simulink model "excercise1_tf2"  (R2023b)
settings: Solver=VariableStepAuto  StartTime=0.0  StopTime=100  RelTol=1e-3
undefined symbols (not defined in the file): d, m
settings Model: Creator=elliot  LastModifiedBy=elliot

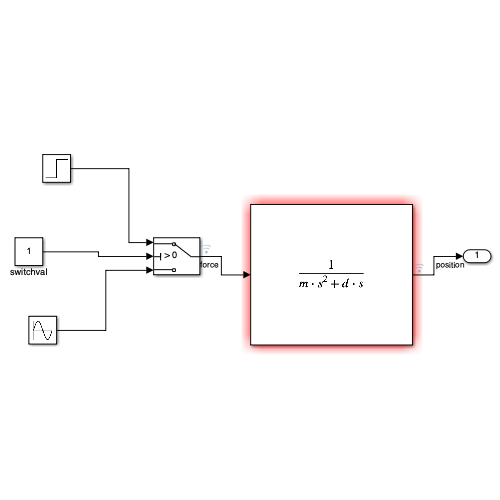
[thumbnail: Simulink's stored preview of the top-level diagram]
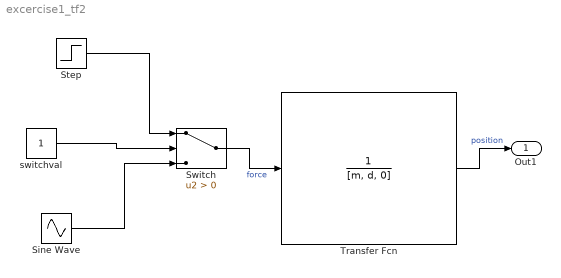
== system excercise1_tf2 ==
  Sine Wave : Sin  SampleTime=0
  Step : Step  Time=0  SampleTime=0
  Switch : Switch  Criteria=u2 > Threshold  SaturateOnIntegerOverflow=off  InputSameDT=off
  Transfer Fcn : TransferFcn  Denominator=[m, d, 0]
  switchval : Constant
  Out1 : Outport
  wires:
  Transfer Fcn/1 -> Out1/1  "position"
  Switch/1 -> Transfer Fcn/1  "force"
  Step/1 -> Switch/1
  Sine Wave/1 -> Switch/3
  switchval/1 -> Switch/2
